simulink model "load_pos_sensor"  (R2023a)
settings: configuration reference "config" (kept outside this file)
model workspace (MAT data in the model file):
  timer_s = Simulink.Signal
  timer_s.Description = '时间计数器 s'
  timer_s.DataType = 'single'
  timer_s.Dimensions = -1
  timer_s.DimensionsMode = 'auto'
  timer_s.Complexity = 'auto'
  timer_s.SampleTime = -1
  timer_s.SamplingMode = 'auto'
  timer_s.InitialValue = '0'
settings Model: DataDictionary=model_config.sldd  Creator=huangcheng  LastModifiedBy=Administrator
settings ConfigSetRef: SourceName=config

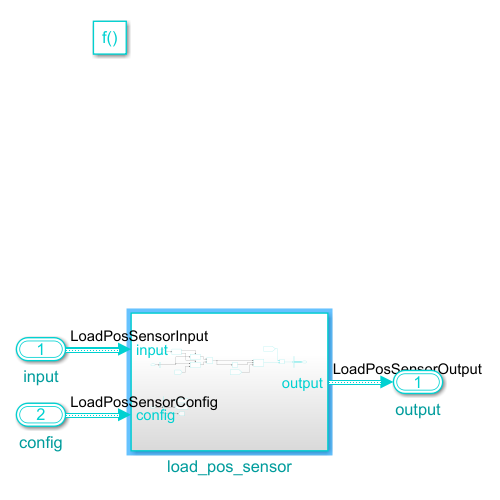
[thumbnail: Simulink's stored preview of the top-level diagram]
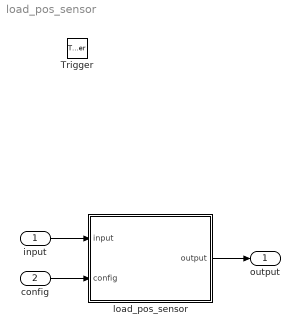
== system load_pos_sensor ==
  input : Inport  OutDataTypeStr=Bus: LoadPosSensorInput  BusOutputAsStruct=on
  config : Inport  Port=2  OutDataTypeStr=Bus: LoadPosSensorConfig  BusOutputAsStruct=on
  Trigger : TriggerPort  TriggerType=function-call  VariantControl=(inherit)  PortDimensions=1
  load_pos_sensor : Subsystem
  output : Outport  OutDataTypeStr=Bus: LoadPosSensorOutput  BusOutputAsStruct=on
  wires:
  input/1 -> load_pos_sensor/1(input)
  config/1 -> load_pos_sensor/2(config)
  load_pos_sensor/1(output) -> output/1

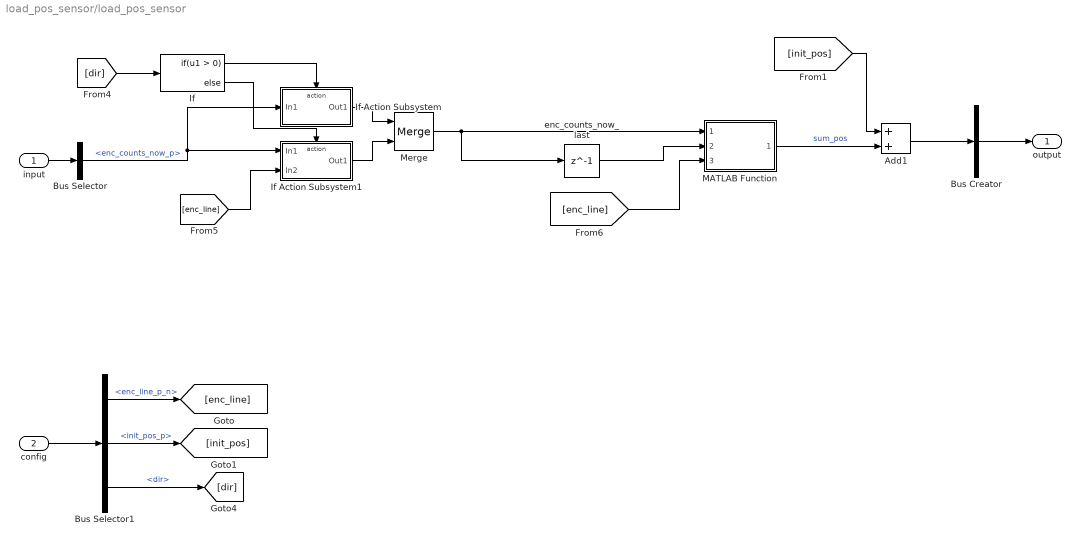
== system load_pos_sensor/load_pos_sensor ==
  input : Inport
  config : Inport  Port=2
  Add1 : Sum
  Bus Creator : BusCreator  Inputs=1  OutDataTypeStr=Bus: LoadPosSensorOutput  NonVirtualBus=on
      settings: InheritFromInputs=off
  Bus Selector : BusSelector  OutputSignals=enc_counts_now_p
  Bus Selector1 : BusSelector  OutputSignals=enc_line_p_n,init_pos_p,dir
  If : If
  If Action Subsystem : Subsystem  TreatAsAtomicUnit=on
  If Action Subsystem1 : Subsystem  TreatAsAtomicUnit=on
  MATLAB Function : MATLAB Function  TreatAsAtomicUnit=on
  Merge : Merge
  enc_counts_now_last : Delay  DelayLength=1  StateName=enc_counts_now_last
  output : Outport
  wires:
  input/1 -> Bus Selector/1
  config/1 -> Bus Selector1/1
  Merge/1 -> enc_counts_now_last/1, MATLAB Function/1(pos_now)
  Bus Selector1/1 -> [enc_line]  "<enc_line_p_n>"
  Bus Selector1/2 -> [init_pos]  "<init_pos_p>"
  Bus Creator/1 -> output/1
  Bus Selector1/3 -> [dir]  "<dir>"
  [dir] -> If/1
  If/1 -> If Action Subsystem/Action
  If/2 -> If Action Subsystem1/Action
  Bus Selector/1 -> If Action Subsystem1/1(In1), If Action Subsystem/1(In1)  "<enc_counts_now_p>"
  If Action Subsystem/1(Out1) -> Merge/1
  If Action Subsystem1/1(Out1) -> Merge/2
  [enc_line] -> If Action Subsystem1/2(In2)
  enc_counts_now_last/1 -> MATLAB Function/2(pos_now_last)
  [enc_line] -> MATLAB Function/3(enc_line)
  [init_pos] -> Add1/1
  Add1/1 -> Bus Creator/1
  MATLAB Function/1(sum_pos) -> Add1/2  "sum_pos"

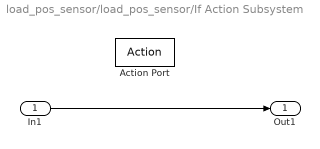
== system load_pos_sensor/load_pos_sensor/If Action Subsystem ==
  In1 : Inport
  Action Port : ActionPort  ActionPortLabel=if(u1 > 0)
  Out1 : Outport
  wires:
  In1/1 -> Out1/1

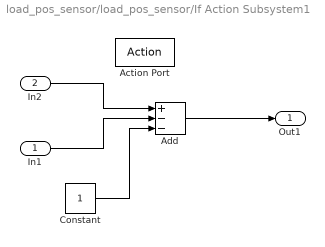
== system load_pos_sensor/load_pos_sensor/If Action Subsystem1 ==
  In1 : Inport
  In2 : Inport  Port=2
  Action Port : ActionPort  ActionPortLabel=else
  Add : Sum  Inputs=+--
  Constant : Constant  OutDataTypeStr=uint32
  Out1 : Outport
  wires:
  In2/1 -> Add/1
  In1/1 -> Add/2
  Add/1 -> Out1/1
  Constant/1 -> Add/3

== matlab function load_pos_sensor/MATLAB Function ==
  data: pos_now input; pos_now_last input; sum_pos output; enc_line input
function sum_pos = fcn(pos_now, pos_now_last, enc_line)

persistent circle_int_n_;

if  isempty(circle_int_n_)
    circle_int_n_ = int64(0);
end
sum_pos = int64(0);
enc_line_half = enc_line / uint32(2);

if pos_now > pos_now_last
    if (pos_now - pos_now_last) > enc_line_half   %向下溢出
        circle_int_n_ = circle_int_n_ - int64(enc_line);  %累计圈数 -1
    end
end

if pos_now < pos_now_last
    if (pos_now_last - pos_now) > enc_line_half   %向上溢出
        circle_int_n_ = circle_int_n_ + int64(enc_line);  %累计圈数 +1
    end
end


sum_pos = circle_int_n_ + int64(pos_now);
